simulink library "quantization"  (R2022a)
settings: Solver=VariableStepAuto  StartTime=0.0  StopTime=10.0  RelTol=1e-3
settings Model: Creator=mcobb  LastModifiedBy=lhill8
settings SolverCC: AlgebraicLoopSolver=TrustRegion
settings DebuggingCC: UnconnectedInputMsg=warning  UnconnectedOutputMsg=warning  UnconnectedLineMsg=warning  SFMachineParentedDataDiag=warning  ArithmeticOperatorsInVariantConditions=warning
settings SFSimCC: CustomCodeUndefinedFunction=UseInterfaceOnly

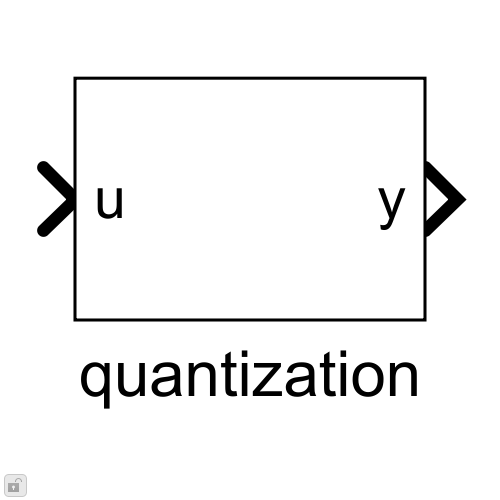
[thumbnail: Simulink's stored preview of the top-level diagram]
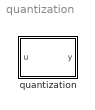
== system quantization ==
  quantization : Subsystem  mask{qnt=0}
      mask prompts: qnt "SNS.quantization object"

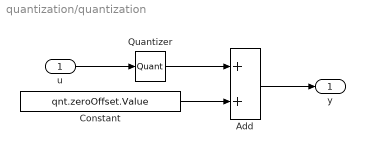
== system quantization/quantization ==
  u : Inport
  Add : Sum
  Constant : Constant  Value=qnt.zeroOffset.Value
  Quantizer : Quantizer  QuantizationInterval=qnt.stepSize.Value
  y : Outport  VectorParamsAs1DForOutWhenUnconnected=off
  wires:
  u/1 -> Quantizer/1
  Quantizer/1 -> Add/1
  Add/1 -> y/1
  Constant/1 -> Add/2
